simulink model "Simulacao_Exemplo_04_Fuzzy_v2"  (R2016a)
settings: Solver=ode45  StartTime=0.0  StopTime=235  FixedStep=0.1  MaxStep=5e-1  RelTol=1e-1
libraries: simulink x6, fuzblock x1
settings Model: Creator=MeneghettiAir  LastModifiedBy=Larisse Rodrigues
settings SolverCC: ZeroCrossControl=DisableAll
settings DataIOCC: LimitDataPoints=on  SaveFormat=Array
settings DebuggingCC: MaxConsecutiveZCsMsg=none  SolverPrmCheckMsg=warning
settings HardwareCC: ProdBitPerPointer=32  ProdLargestAtomicFloat=None  ProdIntDivRoundTo=Undefined  ProdEndianess=Unspecified  ProdWordSize=32  ProdHWDeviceType=32-bit Generic
settings ModelReferenceCC: PropagateSignalLabelsOutOfModel=off
settings ConfigComp: CovModelRefEnable=Off  CovSFcnEnable=off

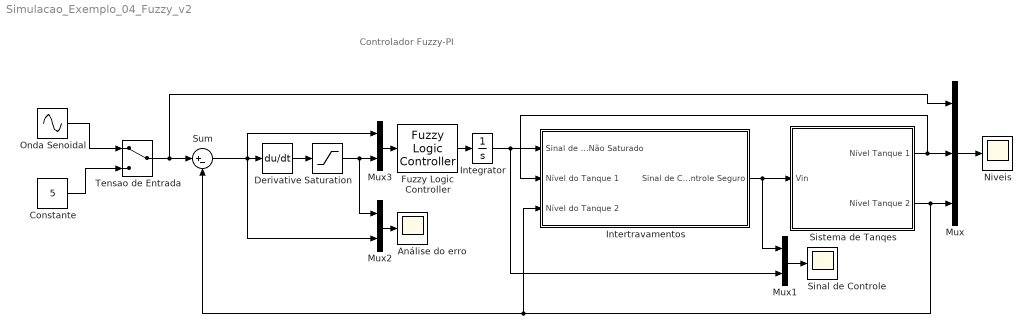
== system Simulacao_Exemplo_04_Fuzzy_v2 ==
  note: Controlador Fuzzy-PI
  Análise do erro : Scope
  Constante : Constant  Value=5
  Derivative : Derivative
  Fuzzy Logic Controller : fuzblock/Fuzzy Logic  Controller  fis='C:\Users\Larisse Rodrigues\Downloads\Simulacao_Exemplo_04_Fuzzy_v2.slx\controle_fuzzy4.fis'
  Integrator : Integrator  ZeroCross=off
  Intertravamentos : Subsystem
  Mux : Mux  Inputs=3
  Mux1 : Mux  Inputs=2
  Mux2 : Mux  Inputs=2
  Mux3 : Mux  Inputs=2
  Niveis : Scope
  Onda Senoidal : Sin  Amplitude=2  Bias=2  Frequency=0.2  SampleTime=0
  Saturation : Saturate  UpperLimit=1  LowerLimit=-1  ZeroCross=off
  Sinal de Controle : Scope
  "Sistema de Tanqes " : Subsystem
  Sum : Sum  Inputs=|+-
  Tensao de Entrada : ManualSwitch
  wires:
  Mux/1 -> Niveis/1
  Tensao de Entrada/1 -> Sum/1, Mux/1
  Constante/1 -> Tensao de Entrada/2
  Onda Senoidal/1 -> Tensao de Entrada/1
  "Sistema de Tanqes "/2(Nível Tanque 2) -> Intertravamentos/3(Nível do Tanque 2), Sum/2, Mux/3
  "Sistema de Tanqes "/1(Nível Tanque 1) -> Intertravamentos/2(Nível do Tanque 1), Mux/2
  Mux1/1 -> Sinal de Controle/1
  Intertravamentos/1(Sinal de Controle Seguro) -> "Sistema de Tanqes "/1(Vin), Mux1/1
  Integrator/1 -> Intertravamentos/1(Sinal de Controle Não Saturado), Mux1/2
  Mux2/1 -> Análise do erro/1
  Mux3/1 -> Fuzzy Logic Controller/1
  Saturation/1 -> Mux2/1, Mux3/2
  Derivative/1 -> Saturation/1
  Sum/1 -> Mux3/1, Derivative/1, Mux2/2
  Fuzzy Logic Controller/1 -> Integrator/1

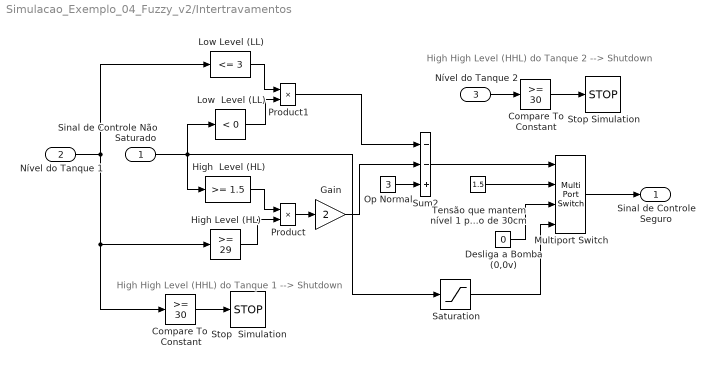
== system Simulacao_Exemplo_04_Fuzzy_v2/Intertravamentos ==
  note: High High Level (HHL) do Tanque 2 --> Shutdown
  note: High High Level (HHL) do Tanque 1 --> Shutdown
  Sinal de Controle Não Saturado : Inport
  Nível do Tanque 1 : Inport  Port=2
  Nível do Tanque 2 : Inport  Port=3
  Compare To  Constant : simulink/Logic and Bit Operations/Compare To Constant  relop=>=  const=30  OutDataTypeStr=boolean
  Compare To Constant : simulink/Logic and Bit Operations/Compare To Constant  relop=>=  const=30  OutDataTypeStr=boolean
  Desliga a Bomba (0,0v) : Constant  Value=0
  Gain : Gain  Gain=2
  High  Level (HL) : simulink/Logic and Bit Operations/Compare To Constant  relop=>=  const=1.5  OutDataTypeStr=uint8
  "High Level (HL)   " : simulink/Logic and Bit Operations/Compare To Constant  relop=>=  const=29  OutDataTypeStr=uint8
  Low  Level (LL) : simulink/Logic and Bit Operations/Compare To Constant  relop=<  const=0  OutDataTypeStr=uint8
  Low Level (LL) : simulink/Logic and Bit Operations/Compare To Constant  relop=<=  const=3  OutDataTypeStr=uint8
  Multiport Switch : MultiPortSwitch
  Op Normal : Constant  Value=3
  Product : Product
  Product1 : Product
  Saturation : Saturate  UpperLimit=4  LowerLimit=-4
  Stop  Simulation : Stop
  Stop Simulation : Stop
  Sum2 : Sum  Inputs=--+
  Tensão que mantem nível 1 próximo de 30cm : Constant  Value=1.5
  Sinal de Controle Seguro : Outport
  wires:
  Sinal de Controle Não Saturado/1 -> Saturation/1, Low  Level (LL)/1, High  Level (HL)/1
  Desliga a Bomba (0,0v)/1 -> Multiport Switch/3
  Tensão que mantem nível 1 próximo de 30cm/1 -> Multiport Switch/2
  Saturation/1 -> Multiport Switch/4
  Sum2/1 -> Multiport Switch/1
  Multiport Switch/1 -> Sinal de Controle Seguro/1
  Nível do Tanque 1/1 -> Low Level (LL)/1, Compare To  Constant/1, "High Level (HL)   "/1
  High  Level (HL)/1 -> Product/1
  "High Level (HL)   "/1 -> Product/2
  Low Level (LL)/1 -> Product1/1
  Low  Level (LL)/1 -> Product1/2
  Product1/1 -> Sum2/1
  Op Normal/1 -> Sum2/3
  Product/1 -> Gain/1
  Gain/1 -> Sum2/2
  Compare To Constant/1 -> Stop Simulation/1
  Nível do Tanque 2/1 -> Compare To Constant/1
  Compare To  Constant/1 -> Stop  Simulation/1

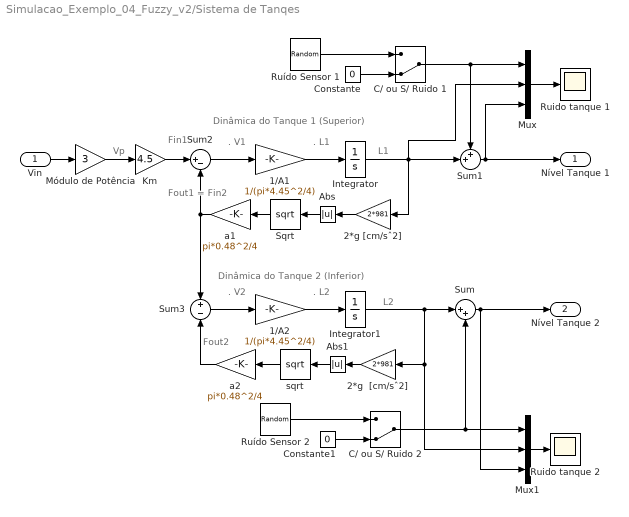
== system Simulacao_Exemplo_04_Fuzzy_v2/Sistema de Tanqes  ==
  note: Dinâmica do Tanque 1 (Superior)
  note: L1
  note: Fin1
  note: Fout1
      | =
      | Fin2
  note: .
      | L1
  note: .
      | V1
  note: L2
  note: Fout2
  note: .
      | L2
  note: .
      | V2
  note: Dinâmica do Tanque 2 (Inferior)
  note: Vp
  Vin : Inport
  1/A1 : Gain  Gain=1/(pi*4.45^2/4)
  1/A2 : Gain  Gain=1/(pi*4.45^2/4)
  2*g  [cm/sˆ2] : Gain  Gain=2*981
  2*g [cm/sˆ2] : Gain  Gain=2*981
  Abs : Abs
  Abs1 : Abs
  C/ ou S/ Ruido 1 : ManualSwitch  CurrentSetting=0
  C/ ou S/ Ruido 2 : ManualSwitch  CurrentSetting=0
  Constante : Constant  Value=0
  Constante1 : Constant  Value=0
  Integrator : Integrator  UpperSaturationLimit=100  LowerSaturationLimit=0  ZeroCross=off
  Integrator1 : Integrator  UpperSaturationLimit=100  LowerSaturationLimit=0
  Km : Gain  Gain=4.5
  Mux : Mux  Inputs=3
  Mux1 : Mux  Inputs=3
  Módulo de Potência : Gain  Gain=3
  Ruido tanque 1 : Scope
  Ruido tanque 2 : Scope
  Ruído Sensor 1 : UniformRandomNumber  Minimum=-0.1  Maximum=0.1  Seed=round(rand(1)*100)  SampleTime=0.5
  Ruído Sensor 2 : UniformRandomNumber  Minimum=-0.1  Maximum=0.1  Seed=round(rand(1)*100)  SampleTime=0.7
  Sqrt : Sqrt  SaturateOnIntegerOverflow=on
  Sum : Sum  Inputs=|++
  Sum1 : Sum  Inputs=++|
  Sum2 : Sum  Inputs=|+-
  Sum3 : Sum  Inputs=+-
  a1 : Gain  Gain=pi*0.48^2/4
  a2 : Gain  Gain=pi*0.48^2/4
  sqrt : Sqrt  SaturateOnIntegerOverflow=on
  Nível Tanque 1 : Outport
  Nível Tanque 2 : Outport  Port=2
  wires:
  Vin/1 -> Módulo de Potência/1
  Sum/1 -> Nível Tanque 2/1, Mux1/3
  Mux/1 -> Ruido tanque 1/1
  Mux1/1 -> Ruido tanque 2/1
  Sum1/1 -> Nível Tanque 1/1, Mux/3
  C/ ou S/ Ruido 1/1 -> Mux/1, Sum1/1
  C/ ou S/ Ruido 2/1 -> Sum/2, Mux1/1
  2*g [cm/sˆ2]/1 -> Abs/1
  Sqrt/1 -> a1/1
  Km/1 -> Sum2/1
  a1/1 -> Sum2/2, Sum3/1
  Sum2/1 -> 1/A1/1
  1/A1/1 -> Integrator/1
  2*g  [cm/sˆ2]/1 -> Abs1/1
  sqrt/1 -> a2/1
  Sum3/1 -> 1/A2/1
  1/A2/1 -> Integrator1/1
  a2/1 -> Sum3/2
  Módulo de Potência/1 -> Km/1
  Integrator/1 -> Sum1/2, Mux/2, 2*g [cm/sˆ2]/1
  Integrator1/1 -> Mux1/2, 2*g  [cm/sˆ2]/1, Sum/1
  Ruído Sensor 1/1 -> C/ ou S/ Ruido 1/1
  Constante/1 -> C/ ou S/ Ruido 1/2
  Ruído Sensor 2/1 -> C/ ou S/ Ruido 2/1
  Constante1/1 -> C/ ou S/ Ruido 2/2
  Abs/1 -> Sqrt/1
  Abs1/1 -> sqrt/1
